simulink model "simulink_model_test"  (R2016a)
settings: Solver=ode23tb  StartTime=1  StopTime=27622  MaxStep=1  RelTol=1e-4
undefined symbols (not defined in the file or in its folder): Ion, Lithium
libraries: powerlib x2, electricdrivelib x1
Description:
  | Copyright 2008-2016 The MathWorks, Inc.
settings Model: NumberOfSteps=100  Creator=MathWorks  LastModifiedBy=fkazhami
settings DataIOCC: LimitDataPoints=on  SaveFormat=Array
settings OptimizationCC: ExpressionDepthLimit=2147483647  InitFltsAndDblsToZero=on
settings DebuggingCC: UnderspecifiedInitializationDetection=Classic  MergeDetectMultiDrivingBlocksExec=none  SignalResolutionControl=TryResolveAllWithWarning  SolverPrmCheckMsg=warning  FcnCallInpInsideContextMsg=UseLocalSettings  AllowSymbolicDim=off  StateNameClashWarn=warning
settings HardwareCC: ProdBitPerPointer=32  ProdLargestAtomicFloat=None  ProdIntDivRoundTo=Undefined  ProdEndianess=Unspecified  ProdWordSize=32  ProdHWDeviceType=32-bit Generic
settings ModelReferenceCC: PropagateSignalLabelsOutOfModel=off
settings GRTTargetCC: CombineOutputUpdateFcns=off  GRTInterface=on
settings ConfigComp: CovModelRefEnable=Off

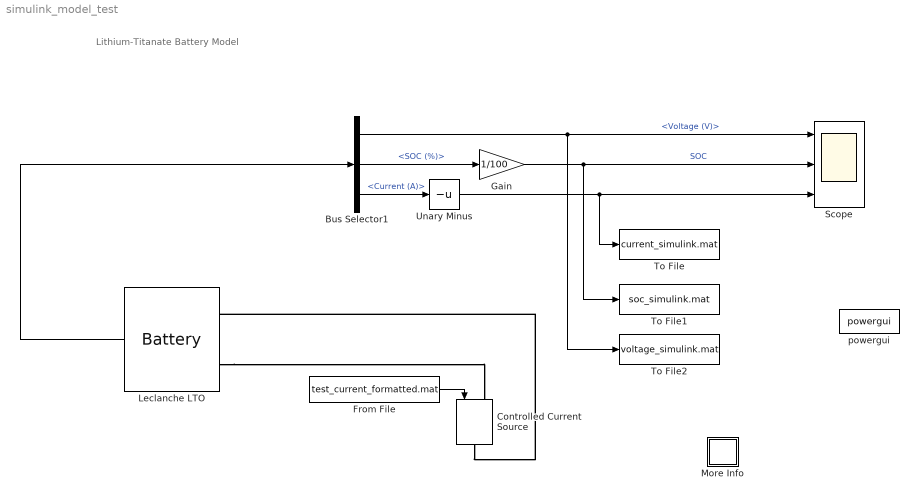
== system simulink_model_test ==
  note: Lithium-Titanate Battery Model
  Bus Selector1 : BusSelector  OutputSignals=Voltage (V),SOC (%),Current (A)
  Controlled Current Source : powerlib/Electrical Sources/Controlled Current Source  Initialize=on  Source_Type=DC  Amplitude=0  Phase=0  Frequency=0  Measurements=None
  From File : FromFile  FileName=test_current_formatted.mat  SampleTime=10
  Gain : Gain  Gain=1/100
  Leclanche LTO : electricdrivelib/Extra Sources/Battery  BatType=Lithium-Ion  ShowTempParam=off  ThermalPreset=no  NomV=1.95  NomQ=30  SOC=11.1  Batt_Tr=30  PresetModel=off  MaxQ=32  MinV=1.5  FullV=2.7  Dis_rate=30  R=0.002  Normal_OP=25  expZone="[2.5      1]"  current=[50 100 150]  Units=Ampere-hour  Tci=20  NomT=25  T2=0  MaxQ2=2.208  FullV2=3.45  Normal_OP2=2.8  expZone2="[3.22        0.23]"  Rca=0.6  ti=1000  Dp=0
  More Info : Subsystem
      settings: OpenFcn=showdemo(bdroot(gcb))
      mask Display: disp('?')
  Scope : Scope  NumInputPorts=3
  To File : ToFile  Filename=current_simulink.mat  MatrixName=c  SampleTime=1
  To File1 : ToFile  Filename=soc_simulink.mat  MatrixName=soc  SampleTime=1
  To File2 : ToFile  Filename=voltage_simulink.mat  MatrixName=v  SampleTime=1
  Unary Minus : UnaryMinus
  powergui : powerlib/powergui  SimulationMode=Discrete  SolverType=Tustin  SampleTime=1  frequency=60  SPID=off  DisableSnubberDevices=off  DisableRonSwitches=off  DisableVfSwitches=off  SwTol=0  DisplayEquations=off  Interpol=off  ExternalGateDelay=off  methode=off  Ts=0  FunctionMessages=off  echomessages=off  HookPort=off  EnableUseOfTLC=off  x0status=blocks  frequencyindice=0  Pbase=100e6  ErrMax=1e-4  Iterations=50  UnitsV=V  UnitsW=W  buscounter=0  RestoreLinks=warning  ResistiveCurrentMeasurement=off  Frange=[0:2:500]  Ylog=off  Xlog=on  ShowGrid=off  save=off  variable=ZData  structure=0  ZoomFFT=on  StartTime=0.0  cycles=1  DisplayStyle=1  fundamental=60  FreqAxis=off  MaxFrequency=1000  frequencyindicesteady=1  RmsSteady=1  display=off
  wires:
  Leclanche LTO/1 -> Bus Selector1/1
  Bus Selector1/2 -> Gain/1  "<SOC (%)>"
  Gain/1 -> To File1/1, Scope/2  "SOC"
  Bus Selector1/3 -> Unary Minus/1  "<Current (A)>"
  From File/1 -> Controlled Current Source/1
  Unary Minus/1 -> To File/1, Scope/3
  Bus Selector1/1 -> To File2/1, Scope/1  "<Voltage (V)>"
  connections:
  Leclanche LTO/LConn2 -- Controlled Current Source/LConn1
  Controlled Current Source/RConn1 -- Leclanche LTO/LConn1

== system simulink_model_test/More Info ==
